simulink library "Start_Delay"  (R2018b)
settings: Solver=ode45  StartTime=0.0  StopTime=10.0  RelTol=1e-3  EnableMultiTasking=on
libraries: simulink x1
settings Model: Creator=lena.frank  LastModifiedBy=P41573
settings DataIOCC: LimitDataPoints=on  SaveFormat=Array  SignalLoggingSaveFormat=ModelDataLogs
settings OptimizationCC: ExpressionDepthLimit=2147483647  LifeSpan=inf
settings DebuggingCC: UnderspecifiedInitializationDetection=Classic  MergeDetectMultiDrivingBlocksExec=none  SolverPrmCheckMsg=warning  FcnCallInpInsideContextMsg=warning  StateNameClashWarn=warning  SFUnexpectedBacktrackingDiag=warning  SFNoUnconditionalDefaultTransitionDiag=warning  SFExecutionAtInitializationDiag=none
settings HardwareCC: ProdBitPerPointer=32  ProdBitPerSizeT=32  ProdBitPerPtrDiffT=32  ProdLargestAtomicFloat=None  ProdIntDivRoundTo=Undefined  ProdEndianess=Unspecified  ProdWordSize=32  ProdHWDeviceType=32-bit Generic
settings ModelReferenceCC: PropagateSignalLabelsOutOfModel=off
settings SFSimCC: SimUseLocalCustomCode=off
settings RTWCC: RTWUseLocalCustomCode=off
settings CodeAppCC: StateflowObjectComments=on
settings GRTTargetCC: TargetLangStandard=C89/C90 (ANSI)  GeneratePreprocessorConditionals=Disable all  CombineOutputUpdateFcns=off  GRTInterface=on
settings ConfigComp: CovMetricSettings=dw  CovHtmlReporting=on  CovSaveCumulativeToWorkspaceVar=on  CovSaveSingleToWorkspaceVar=on  CovExternalEMLEnable=off

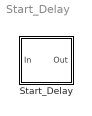
== system Start_Delay ==
  Start_Delay : Subsystem  mask(Start Delay){tstartdelay=5}
      mask prompts: tstartdelay "Start delay time in s"
      mask help: The output is delayed for the delay time, than it equal to the input.
      mask Help: web(fullfile(path_carnot('help'),'Start_Delay.html'),'-helpbrowser')
      mask Display:
      | plot(-20,-30,120,100,[10,20,40,60,80,90,90,80,60,40,20,10,10],[40,20,10,10,20,40,60,80,90,90,80,60,40],[55,46],[95,95],[50,50],[90,95],[50,50,24],[88,50,66],[10,13],[50,50],[90,87],[50,50],[50,50],[10,15])
      | disp('\n\nDelay On')

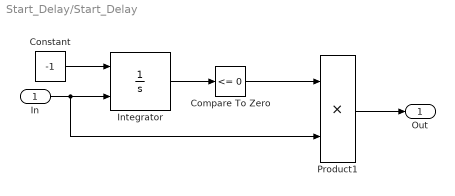
== system Start_Delay/Start_Delay ==
  In : Inport
  Compare To Zero : simulink/Logic and Bit Operations/Compare To Zero  relop=<=  OutDataTypeStr=uint8
  Constant : Constant  Value=-1
  Integrator : Integrator  ExternalReset=rising  InitialCondition=tstartdelay  LimitOutput=on  LowerSaturationLimit=0
  Product1 : Product  RndMeth=Zero
  Out : Outport
  wires:
  Product1/1 -> Out/1
  In/1 -> Integrator/2, Product1/2
  Compare To Zero/1 -> Product1/1
  Integrator/1 -> Compare To Zero/1
  Constant/1 -> Integrator/1
